simulink model "regulator_pid"  (R2013a)
settings: Solver=ode45  StartTime=0.0  StopTime=10.0  MaxStep=0.01  RelTol=1e-3
values from neighbouring files (symbols this model uses):
  k1 = 3    [skrypt_pid.m]
  k2 = 2    [skrypt_pid.m]
  Td = 1.5    [skrypt_pid.m]
  Tp = 0.1    [skrypt_pid.m]
  x = 0    [skrypt_pid.m]
settings Model: Creator=L13-3  LastModifiedBy=Dawid Perdek
settings DataIOCC: SignalLoggingSaveFormat=ModelDataLogs
settings DebuggingCC: UnderspecifiedInitializationDetection=Simplified  MultiTaskDSMMsg=warning  MultiTaskCondExecSysMsg=none  StateNameClashWarn=none  StrictBusMsg=ErrorOnBusTreatedAsVector  NonBusSignalsTreatedAsBus=error
settings RTWCC: IncludeERTFirstTime=on
settings GRTTargetCC: CodeReplacementLibrary=None  CPPClassGenCompliant=on

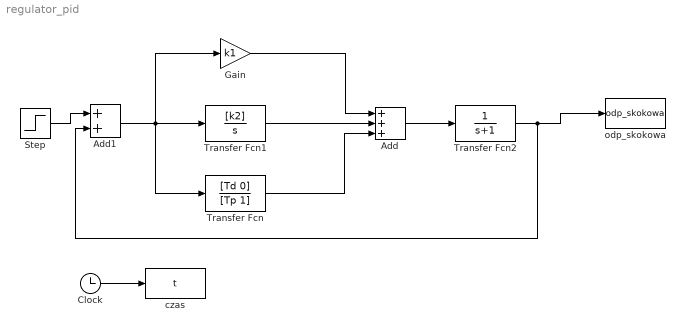
== system regulator_pid ==
  Add : Sum  Inputs=+++
  Add1 : Sum
  Clock : Clock
  Gain : Gain  Gain=k1
  Step : Step  Time=x  SampleTime=0
  Transfer Fcn : TransferFcn  Numerator=[Td 0]  Denominator=[Tp 1]
  Transfer Fcn1 : TransferFcn  Numerator=[k2]  Denominator=[1 0]
  Transfer Fcn2 : TransferFcn  Denominator=[1 1]
  czas : ToWorkspace  VariableName=t  SampleTime=-1
  odp_skokowa : ToWorkspace  VariableName=odp_skokowa  SampleTime=-1
  wires:
  Gain/1 -> Add/1
  Clock/1 -> czas/1
  Transfer Fcn/1 -> Add/3
  Transfer Fcn1/1 -> Add/2
  Transfer Fcn2/1 -> Add1/2, odp_skokowa/1
  Add/1 -> Transfer Fcn2/1
  Step/1 -> Add1/1
  Add1/1 -> Transfer Fcn/1, Gain/1, Transfer Fcn1/1
